simulink model "theecontrol2"  (R2021a)
settings: Solver=VariableStepAuto  StartTime=0.0  StopTime=2  RelTol=1e-3
libraries: spsIGBTDiodeLib x6, spsDCVoltageSourceLib x1, spsGroundLib x1, spsThreePhaseSeriesRLCBranchLib x1, spsThreePhaseVIMeasurementLib x1, spsTriangleGeneratorLib x1, spspowerguiLib x1
settings Model: Creator=Asus  LastModifiedBy=User
settings SolverCC: AlgebraicLoopSolver=TrustRegion
settings DebuggingCC: ArithmeticOperatorsInVariantConditions=warning
settings SFSimCC: CustomCodeUndefinedFunction=UseInterfaceOnly

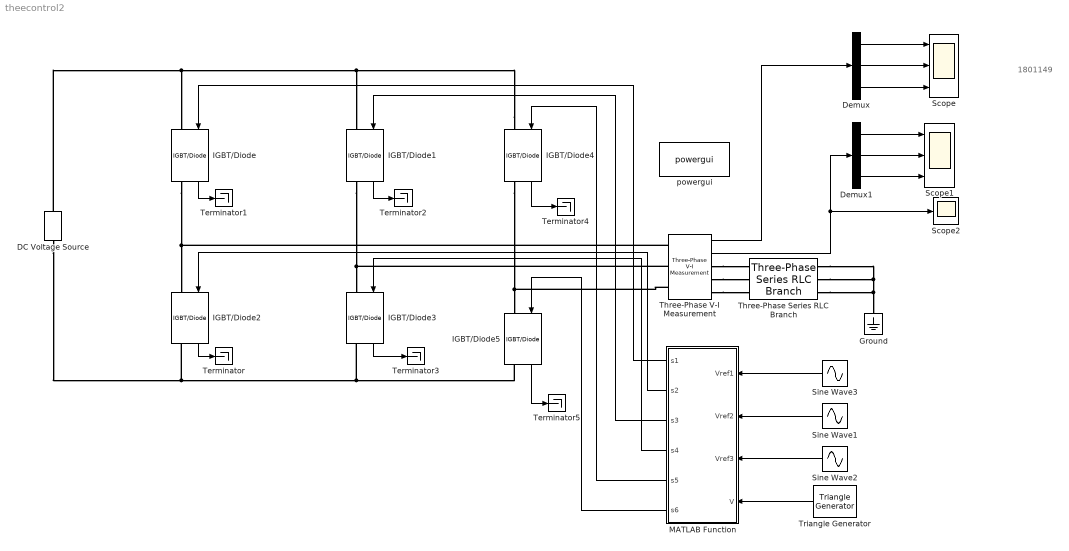
== system theecontrol2 ==
  note: 1801149
  DC Voltage Source : spsDCVoltageSourceLib/DC Voltage Source  Amplitude=50  Measurements=None
  Demux : Demux  Outputs=3
  Demux1 : Demux  Outputs=3
  Ground : spsGroundLib/Ground  LConnTagsString=a
  IGBT/Diode{,1..5} (6 alike) : spsIGBTDiodeLib/IGBT//Diode  Ron=1e-3  Rs=1e5  Cs=inf  Measurements=on
  MATLAB Function : MATLAB Function  TreatAsAtomicUnit=on
  Scope : Scope  NumInputPorts=3
  Scope1 : Scope  NumInputPorts=3
  Scope2 : Scope
  Sine Wave1 : Sin  Frequency=50*pi*2  Phase=120*pi/180  SampleTime=0
  Sine Wave2 : Sin  Frequency=50*pi*2  Phase=240*pi/180  SampleTime=0
  Sine Wave3 : Sin  Frequency=50*pi*2  SampleTime=0
  Terminator{,1..5} (6 alike) : Terminator
  Three-Phase Series RLC Branch : spsThreePhaseSeriesRLCBranchLib/Three-Phase Series RLC Branch  LConnTagsString=A|B|C  RConnTagsString=A|B|C  BranchType=RL  Resistance=100  Inductance=1000e-3  Capacitance=1e-6  Measurements=None
  Three-Phase V-I Measurement : spsThreePhaseVIMeasurementLib/Three-Phase V-I Measurement  VoltageMeasurement=phase-to-ground  SetLabelV=off  LabelV=Vabc  Vpu=off  VpuLL=off  CurrentMeasurement=yes  SetLabelI=off  LabelI=Iabc  Ipu=off  Pbase=100e6  Vbase=500e3  OutputType=Complex  PhasorSimulation=off  PSBequivalent=0
  Triangle Generator : spsTriangleGeneratorLib/Triangle Generator  Freq=1000  Phase=0  Ts=0
  powergui : spspowerguiLib/powergui  Priority=1  SimulationMode=Discrete  SampleTime=50e-6  frequency=60  Iterations=50  frequencyindice=0  Pbase=100e6  ErrMax=1e-4  UnitsV=kV  UnitsW=MW  buscounter=0  FunctionMessages=off  echomessages=off  EnableUseOfTLC=off  CurrentSourceSwitches=off  DisableSnubberDevices=off  DisableRonSwitches=off  DisableVfSwitches=off  DisplayEquations=off  AutomaticDiscreteSolvers=off  SolverType=Tustin/Backward Euler (TBE)  Interpol=off  ExternalGateDelay=off  methode=off  Ts=100  x0status=blocks  SPID=on  SwTol=0  HookPort=off  NonlinearTolerance=1e-4  nMaxIteration=100  ContinueOnMaxIteration=off  RestoreLinks=warning  ResistiveCurrentMeasurement=off  Frange=[0:2:500]  Ylog=off  Xlog=on  ShowGrid=off  save=off  variable=ZData  structure=0  ZoomFFT=off  StartTime=0.0  cycles=1  DisplayStyle=1  fundamental=60  FreqAxis=off  MaxFrequency=1000  frequencyindicesteady=1  RmsSteady=1  display=off
  wires:
  Sine Wave3/1 -> MATLAB Function/1(Vref1)
  Sine Wave1/1 -> MATLAB Function/2(Vref2)
  Sine Wave2/1 -> MATLAB Function/3(Vref3)
  Triangle Generator/1 -> MATLAB Function/4(V)
  Three-Phase V-I Measurement/1 -> Demux/1
  Three-Phase V-I Measurement/2 -> Demux1/1, Scope2/1
  Demux/1 -> Scope/1
  Demux/2 -> Scope/2
  Demux/3 -> Scope/3
  Demux1/2 -> Scope1/2
  Demux1/1 -> Scope1/1
  Demux1/3 -> Scope1/3
  MATLAB Function/1(s1) -> IGBT/Diode/1
  MATLAB Function/3(s3) -> IGBT/Diode1/1
  MATLAB Function/5(s5) -> IGBT/Diode4/1
  MATLAB Function/2(s2) -> IGBT/Diode2/1
  MATLAB Function/4(s4) -> IGBT/Diode3/1
  MATLAB Function/6(s6) -> IGBT/Diode5/1
  IGBT/Diode2/1 -> Terminator/1
  IGBT/Diode/1 -> Terminator1/1
  IGBT/Diode1/1 -> Terminator2/1
  IGBT/Diode3/1 -> Terminator3/1
  IGBT/Diode4/1 -> Terminator4/1
  IGBT/Diode5/1 -> Terminator5/1
  connections:
  IGBT/Diode4/RConn1 -- Three-Phase V-I Measurement/LConn3 -- IGBT/Diode5/LConn1
  IGBT/Diode5/RConn1 -- DC Voltage Source/LConn1 -- IGBT/Diode2/RConn1 -- IGBT/Diode3/RConn1
  IGBT/Diode/RConn1 -- Three-Phase V-I Measurement/LConn1 -- IGBT/Diode2/LConn1
  IGBT/Diode4/LConn1 -- IGBT/Diode1/LConn1 -- IGBT/Diode/LConn1 -- DC Voltage Source/RConn1
  IGBT/Diode1/RConn1 -- Three-Phase V-I Measurement/LConn2 -- IGBT/Diode3/LConn1
  Three-Phase V-I Measurement/RConn1 -- Three-Phase Series RLC Branch/LConn1
  Three-Phase V-I Measurement/RConn2 -- Three-Phase Series RLC Branch/LConn2
  Three-Phase V-I Measurement/RConn3 -- Three-Phase Series RLC Branch/LConn3
  Three-Phase Series RLC Branch/RConn1 -- Ground/LConn1 -- Three-Phase Series RLC Branch/RConn3 -- Three-Phase Series RLC Branch/RConn2

== matlab function theecontrol2/MATLAB Function ==
  data: Vref1 input; s1 output; Vref2 input; Vref3 input; s2 output; s3 output; s4 output; s5 output; s6 output; V input
function [s1,s2,s3,s4,s5,s6] = fcn(Vref1,Vref2,Vref3,V)
if Vref1 >= 0
   if Vref1 >= V
        s1 = 1;
        s2 = 0;
   else
        s1 = 0;
        s2 = 1;
   end
else
    if Vref1 <= V
        s1 = 0;
        s2 = 1;
   else
        s1 = 1;
        s2 = 0;
   end
end
if Vref2 >= 0
    if Vref2>= V
        s3 = 1;
        s4 = 0;
    else
        s3 = 0;
        s4 = 1;
    end
else
    if Vref2 <= V
        s3 = 0;
        s4 = 1;
    else
        s3 = 1;
        s4 = 0;
    end
end

if Vref3>=0
    if Vref3 >= V
        s5 = 1;
        s6 = 0;
    else
        s5 = 0;
        s6 = 1;
    end
else
    if Vref3 <= V
        s5 = 0;
        s6 = 1;
    else
        s5 = 1;
        s6 = 0;
    end
end
end
